simulink model "avionic"  (R2021b)
settings: Solver=ode1  StartTime=0.0  StopTime=inf  FixedStep=0.02  RelTol=1e-3  EnableMultiTasking=on
libraries: bbblueCommlib x13, svdutilitieslib x6, simulink x6, bbblueBasicLib x4, bbblueSensorLib x2
settings Model: ExtModeTrigDuration=100  Creator=ASUS  LastModifiedBy=ASUS
settings SolverCC: PositivePriorityOrder=on  AutoInsertRateTranBlk=on
settings OptimizationCC: EnhancedBackFolding=on  PassReuseOutputArgsAs=Individual arguments  ZeroExternalMemoryAtStartup=off  ZeroInternalMemoryAtStartup=off  MaxStackSize=64  OptimizeBlockOrder=speed  DifferentSizesBufferReuse=on  OptimizationCustomize=off  EfficientTunableParamExpr=on
settings DebuggingCC: ParameterTunabilityLossMsg=error
settings HardwareCC: ProdBitPerPointer=32  ProdBitPerSizeT=32  ProdBitPerPtrDiffT=32  ProdLargestAtomicInteger=Long  ProdLargestAtomicFloat=Double  ProdWordSize=32  ProdHWDeviceType=ARM Compatible->ARM Cortex
settings SFSimCC: MATLABDynamicMemAlloc=off
settings RTWCC: Description=Embedded Coder  SystemTargetFile=ert.tlc  HardwareBoard=BeagleBone Blue  TLCOptions="-aInlineSetEventsForThisBaseRateFcn=TLC_FALSE -aSuppressMultiTaskScheduler=TLC_FALSE  -aRateBasedStepFcn=0"  TemplateMakefile=ert_default_tmf  Toolchain=GNU GCC BeagleBone Blue
settings CodeAppCC: ForceParamTrailComments=on  IgnoreCustomStorageClasses=off  OperatorAnnotations=on  SimulinkDataObjDesc=on  SFDataObjDesc=on  InsertBlockDesc=on
settings ERTTargetCC: SupportContinuousTime=on  SupportVariableSizeSignals=on

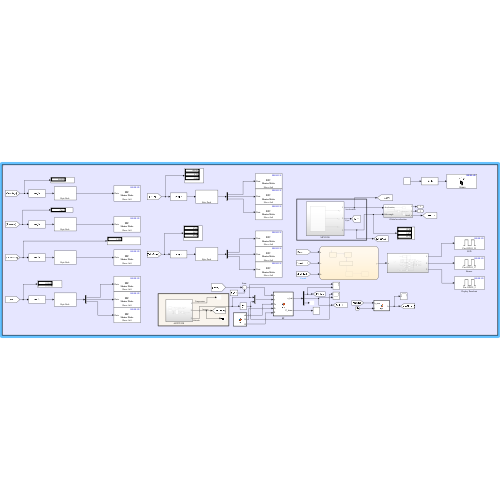
[thumbnail: Simulink's stored preview of the top-level diagram]
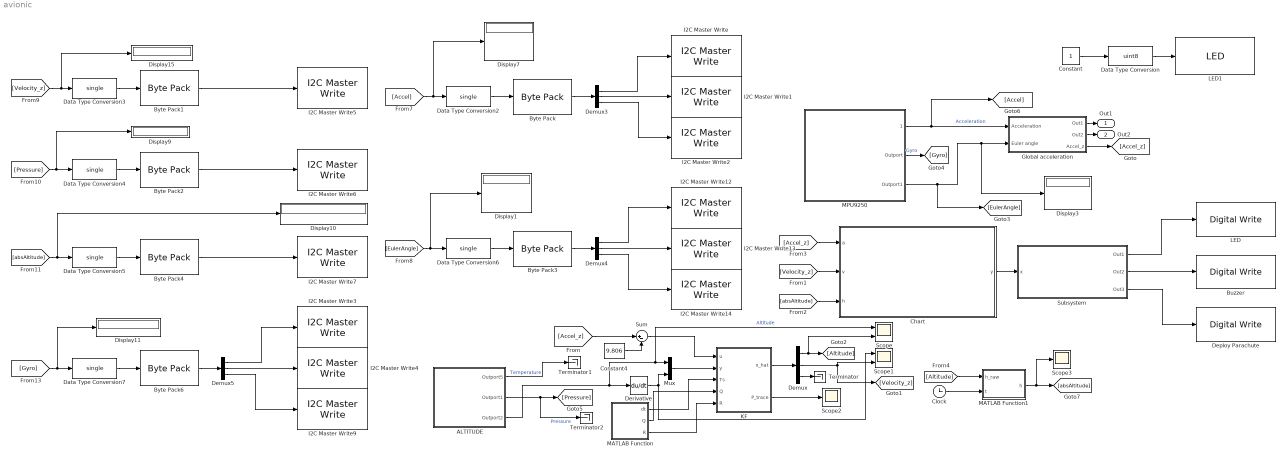
== system avionic ==
  "ALTITUDE " : Subsystem
  "Buzzer " : bbblueBasicLib/Digital Write  GPIOSelect=GPIO1_17  Pin=49  Direction=output
      settings: SourceProductBaseCode=SC_BEAGLEBONE_BLUE
  Byte Pack{,1..4,6} (6 alike) : svdutilitieslib/Byte Pack  maskPackedDataType=uint8  datatypes={'single'}  byteAlign=1  blockPlatform=arduinoert
      settings: SourceProductBaseCode=ANDROID,ARDUINO,ML_ARDUINO,ECCORTEXA,ECCORTEXR,SC_BEAGLEBONE_BLUE,EC_FREEDOM_BOARD,EC_FRDM_K64F,INTEL_BLOCKSET,MICROBIT,NUCLEO,NVIDIA,PX4AUTOPILOTS,RASPPIIO,STMICRODIS,TIC2000,XILINX_BLOCKSET
  Chart : Stateflow chart  TreatAsAtomicUnit=on
  Clock : Clock
  Constant : Constant
  Constant4 : Constant  Value=9.806
  Data Type Conversion : DataTypeConversion  OutDataTypeStr=uint8
  Data Type Conversion{2..7} (6 alike) : DataTypeConversion  OutDataTypeStr=single
  Demux{,3..5} (4 alike) : Demux  Outputs=3
  Deploy Parachute : bbblueBasicLib/Digital Write  GPIOSelect=GPIO3_2  Pin=49  Direction=output
      settings: SourceProductBaseCode=SC_BEAGLEBONE_BLUE
  Derivative : Derivative
  Display{1,3,7,9..11,15} (7 alike) : Display
  Global acceleration : Subsystem
  I2C Master Write{,1..7,9,12..14} (12 alike) : bbblueCommlib/I2C Master Write  I2CModule=1  Mode=Master  SlaveAddress=8  SlaveByteOrder=BigEndian  Direction=Transmitter  RegisterAddressMode=off  RegisterAddress=0  SlaveDataType=uint8  DataLength=1  NoAck=off  RepeatedStart=off  OutputStatus=off
      settings: SourceProductBaseCode=SC_BEAGLEBONE_BLUE
  KF : MATLAB Function  TreatAsAtomicUnit=on
  "LED " : bbblueBasicLib/Digital Write  GPIOSelect=GPIO1_25  Pin=49  Direction=output
      settings: SourceProductBaseCode=SC_BEAGLEBONE_BLUE
  LED1 : bbblueBasicLib/LED  LED=Green
      settings: SourceProductBaseCode=SC_BEAGLEBONE_BLUE
  MATLAB Function : MATLAB Function  TreatAsAtomicUnit=on
  MATLAB Function1 : MATLAB Function  TreatAsAtomicUnit=on
  MPU9250 : Subsystem
  Mux : Mux  Inputs=2
  Scope : Scope  NumInputPorts=2
  Scope1 : Scope  NumInputPorts=2
  Scope2 : Scope
  Scope3 : Scope
  Subsystem : Subsystem
  "Sum " : Sum  Inputs=|+-
  Terminator : Terminator
  Terminator1 : Terminator
  Terminator2 : Terminator
  Out1 : Outport
  Out2 : Outport  Port=2
  wires:
  Demux5/1 -> I2C Master Write3/1
  Subsystem/1(Out1) -> "LED "/1
  MPU9250/1(1) -> [Accel], Global acceleration/1(Acceleration)  "Acceleration"
  Derivative/1 -> Mux/2, Scope1/1
  "ALTITUDE "/3(Outport2) -> Scope/1, Mux/1, Derivative/1  "Altitude"
  [Accel_z] -> "Sum "/1
  "ALTITUDE "/1(Outport5) -> Terminator1/1  "Temperature"
  Data Type Conversion3/1 -> Byte Pack1/1
  Demux3/2 -> I2C Master Write1/1
  Data Type Conversion2/1 -> Byte Pack/1
  Demux4/3 -> I2C Master Write14/1
  Demux3/1 -> I2C Master Write/1
  [Velocity_z] -> Display15/1, Data Type Conversion3/1
  Global acceleration/2(Out2) -> Out2/1
  Byte Pack2/1 -> I2C Master Write6/1
  Demux4/1 -> I2C Master Write12/1
  "ALTITUDE "/2(Outport1) -> [Pressure], Terminator2/1  "Pressure"
  Demux5/2 -> I2C Master Write4/1
  Data Type Conversion6/1 -> Byte Pack3/1
  [Gyro] -> Display11/1, Data Type Conversion7/1
  [EulerAngle] -> Display1/1, Data Type Conversion6/1
  Byte Pack4/1 -> I2C Master Write7/1
  [Velocity_z] -> Chart/2(v)
  Data Type Conversion4/1 -> Byte Pack2/1
  Global acceleration/1(Out1) -> Out1/1
  MPU9250/3(Outport1) -> [EulerAngle], Display3/1, Global acceleration/2(Euler angle)
  Byte Pack1/1 -> I2C Master Write5/1
  Subsystem/3(Out3) -> Deploy Parachute/1
  Data Type Conversion7/1 -> Byte Pack6/1
  Global acceleration/3(Accel_z) -> [Accel_z]
  [absAltitude] -> Display10/1, Data Type Conversion5/1
  Subsystem/2(Out2) -> "Buzzer "/1
  Byte Pack/1 -> Demux3/1
  Demux4/2 -> I2C Master Write13/1
  [Accel_z] -> Chart/1(a)
  [Accel] -> Display7/1, Data Type Conversion2/1
  Demux3/3 -> I2C Master Write2/1
  MPU9250/2(Outport) -> [Gyro]  "Gyro"
  [absAltitude] -> Chart/3(h)
  Chart/1(y) -> Subsystem/1(x)
  Byte Pack3/1 -> Demux4/1
  Byte Pack6/1 -> Demux5/1
  [Pressure] -> Display9/1, Data Type Conversion4/1
  Data Type Conversion5/1 -> Byte Pack4/1
  Demux5/3 -> I2C Master Write9/1
  Data Type Conversion/1 -> LED1/1
  Constant/1 -> Data Type Conversion/1
  Constant4/1 -> "Sum "/2
  "Sum "/1 -> KF/1(u)
  Mux/1 -> KF/2(y)
  MATLAB Function/1(dt) -> KF/3(Ts)
  MATLAB Function/2(Q) -> KF/4(Q)
  MATLAB Function/3(R) -> KF/5(R)
  KF/1(x_hat) -> Demux/1
  KF/2(P_trace) -> Scope2/1
  Demux/1 -> Scope/2, [Altitude]
  Demux/2 -> Scope1/2, [Velocity_z]
  Demux/3 -> Terminator/1
  [Altitude] -> MATLAB Function1/1(h_raw)
  Clock/1 -> MATLAB Function1/2(t)
  MATLAB Function1/1(h) -> Scope3/1, [absAltitude]

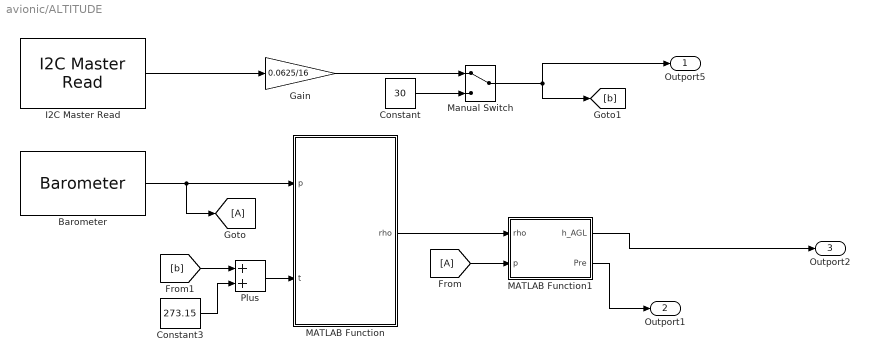
== system avionic/ALTITUDE  ==
  Barometer : bbblueSensorLib/Barometer  OSRSelection=16  IIRFilterCoeff=16  SampleTime=0.02
      settings: SourceProductBaseCode=SC_BEAGLEBONE_BLUE
  Constant : Constant  Value=30
  Constant3 : Constant  Value=273.15
  Gain : Gain  Gain=0.0625/16  OutDataTypeStr=single
  I2C Master Read : bbblueCommlib/I2C Master Read  I2CModule=1  Mode=Master  SlaveAddress=hex2dec('48')  SlaveByteOrder=BigEndian  Direction=Receiver  RegisterAddressMode=off  RegisterAddress=0  SlaveDataType=int16  DataLength=1  NoAck=off  RepeatedStart=off  OutputStatus=off  SampleTime=0.02
      settings: SourceProductBaseCode=SC_BEAGLEBONE_BLUE
  MATLAB Function : MATLAB Function  TreatAsAtomicUnit=on
  MATLAB Function1 : MATLAB Function  TreatAsAtomicUnit=on
  Manual Switch : ManualSwitch
  Plus : Sum
  Outport5 : Outport
  Outport1 : Outport  Port=2
  Outport2 : Outport  Port=3
  wires:
  I2C Master Read/1 -> Gain/1
  Plus/1 -> MATLAB Function/2(t)
  Barometer/1 -> [A], MATLAB Function/1(p)
  Gain/1 -> Manual Switch/1
  MATLAB Function/1(rho) -> MATLAB Function1/1(rho)
  Constant3/1 -> Plus/2
  [A] -> MATLAB Function1/2(p)
  [b] -> Plus/1
  MATLAB Function1/1(h_AGL) -> Outport2/1
  MATLAB Function1/2(Pre) -> Outport1/1
  Constant/1 -> Manual Switch/2
  Manual Switch/1 -> [b], Outport5/1

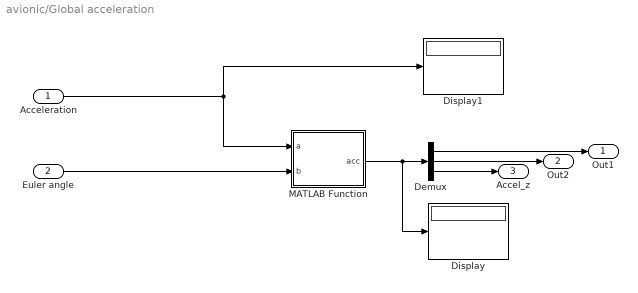
== system avionic/Global acceleration ==
  Acceleration : Inport
  Euler angle : Inport  Port=2
  Demux : Demux  Outputs=3
  Display : Display
  Display1 : Display
  MATLAB Function : MATLAB Function  TreatAsAtomicUnit=on
  Out1 : Outport
  Out2 : Outport  Port=2
  Accel_z : Outport  Port=3
  wires:
  Acceleration/1 -> MATLAB Function/1(a), Display1/1
  MATLAB Function/1(acc) -> Display/1, Demux/1
  Demux/1 -> Out1/1
  Demux/3 -> Accel_z/1
  Euler angle/1 -> MATLAB Function/2(b)
  Demux/2 -> Out2/1

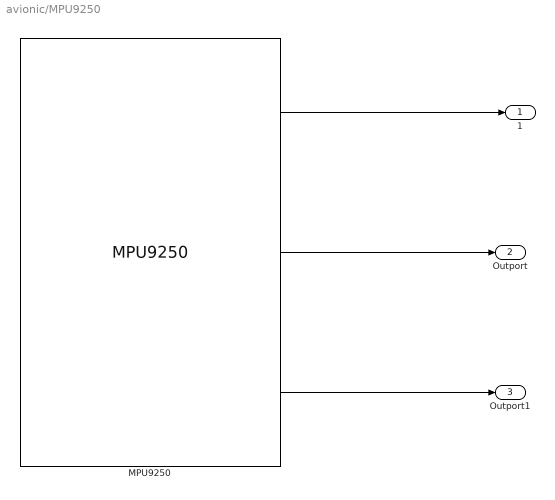
== system avionic/MPU9250 ==
  MPU9250 : bbblueSensorLib/MPU9250  OperationMode=DMP  Accel=on  AngularRate=on  Ak8963Field=off  EulerAngles=on  Quat=off  AccelRange=16G  Acceldlpf=1  GyroRange=250 dps  Gyrodlpf=1  DmpOdr=200 Hz  SampleTime=0.02
      settings: SourceProductBaseCode=SC_BEAGLEBONE_BLUE
  1 : Outport
  Outport : Outport  Port=2
  Outport1 : Outport  Port=3
  wires:
  MPU9250/1 -> 1/1
  MPU9250/2 -> Outport/1
  MPU9250/3 -> Outport1/1

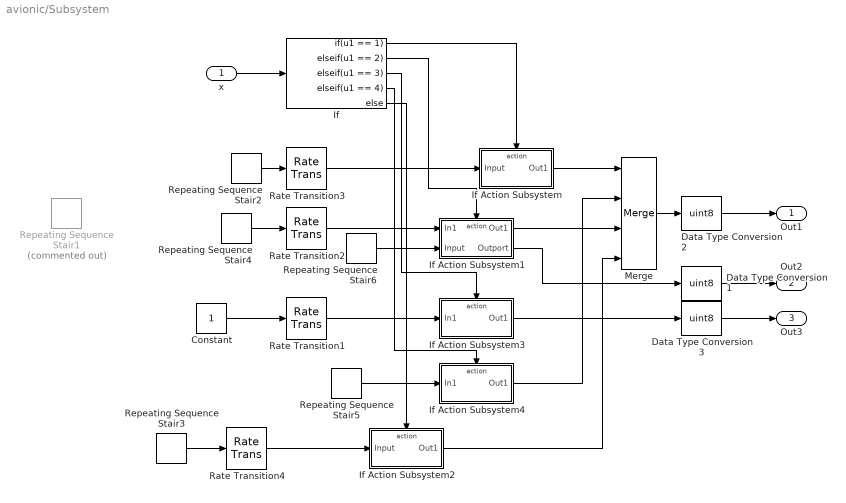
== system avionic/Subsystem ==
  x : Inport
  Constant : Constant
  Data Type Conversion1 : DataTypeConversion  OutDataTypeStr=uint8
  Data Type Conversion2 : DataTypeConversion  OutDataTypeStr=uint8
  Data Type Conversion3 : DataTypeConversion  OutDataTypeStr=uint8
  If : If  IfExpression=u1 == 1  ElseIfExpressions=u1 == 2, u1 == 3, u1 == 4
  If Action Subsystem : Subsystem  TreatAsAtomicUnit=on
  If Action Subsystem1 : Subsystem  TreatAsAtomicUnit=on
  If Action Subsystem2 : Subsystem  TreatAsAtomicUnit=on
  If Action Subsystem3 : Subsystem  TreatAsAtomicUnit=on
  If Action Subsystem4 : Subsystem  TreatAsAtomicUnit=on
  Merge : Merge  Inputs=4
  Rate Transition{1..4} (4 alike) : RateTransition
  Repeating Sequence Stair1 : simulink/Sources/Repeating Sequence Stair  Commented=on  OutValues=[1 0 1 0 0 0 0 0].'  tsamp=0.1  OutMin=[]  OutMax=[]  OutDataTypeStr=double  OutputDataTypeScalingMode=double  OutDataType=fixdt(0,8)  ConRadixGroup=Best Precision: Vector-wise  OutScaling=2^-12
  Repeating Sequence Stair2 : simulink/Sources/Repeating Sequence Stair  OutValues=[1 1 1 1 1 0 0 0 0 0].'  tsamp=0.1  OutMin=[]  OutMax=[]  OutDataTypeStr=double  OutputDataTypeScalingMode=double  OutDataType=fixdt(0,8)  ConRadixGroup=Best Precision: Vector-wise  OutScaling=2^-12
  Repeating Sequence Stair3 : simulink/Sources/Repeating Sequence Stair  OutValues=[1 0 0 0 0 0 0 0 0 0 0 0 0 0 0 0].'  tsamp=0.1  OutMin=[]  OutMax=[]  OutDataTypeStr=double  OutputDataTypeScalingMode=double  OutDataType=fixdt(0,8)  ConRadixGroup=Best Precision: Vector-wise  OutScaling=2^-12
  Repeating Sequence Stair4 : simulink/Sources/Repeating Sequence Stair  OutValues=[1 0 1 0 1 0 0 0].'  tsamp=0.1  OutMin=[]  OutMax=[]  OutDataTypeStr=double  OutputDataTypeScalingMode=double  OutDataType=fixdt(0,8)  ConRadixGroup=Best Precision: Vector-wise  OutScaling=2^-12
  Repeating Sequence Stair5 : simulink/Sources/Repeating Sequence Stair  OutValues=[1 0 1 0 0 0 0 0].'  tsamp=0.1  OutMin=[]  OutMax=[]  OutDataTypeStr=double  OutputDataTypeScalingMode=double  OutDataType=fixdt(0,8)  ConRadixGroup=Best Precision: Vector-wise  OutScaling=2^-12
  Repeating Sequence Stair6 : simulink/Sources/Repeating Sequence Stair  OutValues=[1 0 1 0 1 0 0 0].'  tsamp=0.5  OutMin=[]  OutMax=[]  OutDataTypeStr=double  OutputDataTypeScalingMode=double  OutDataType=fixdt(0,8)  ConRadixGroup=Best Precision: Vector-wise  OutScaling=2^-12
  Out1 : Outport
  Out2 : Outport  Port=2
  Out3 : Outport  Port=3
  wires:
  If/5 -> If Action Subsystem2/Action
  If/1 -> If Action Subsystem/Action
  Repeating Sequence Stair4/1 -> Rate Transition2/1
  Rate Transition2/1 -> If Action Subsystem1/1(In1)
  Merge/1 -> Data Type Conversion2/1
  If Action Subsystem/1(Out1) -> Merge/1
  If Action Subsystem1/1(Out1) -> Merge/3
  If/2 -> If Action Subsystem1/Action
  Data Type Conversion2/1 -> Out1/1
  x/1 -> If/1
  Constant/1 -> Rate Transition1/1
  Rate Transition1/1 -> If Action Subsystem3/1(In1)
  If/3 -> If Action Subsystem3/Action
  If Action Subsystem4/1(Out1) -> Merge/2
  Repeating Sequence Stair5/1 -> If Action Subsystem4/1(In1)
  If/4 -> If Action Subsystem4/Action
  Repeating Sequence Stair2/1 -> Rate Transition3/1
  Rate Transition3/1 -> If Action Subsystem/1(Input)
  Data Type Conversion1/1 -> Out2/1
  Repeating Sequence Stair6/1 -> If Action Subsystem1/2(Input)
  If Action Subsystem1/2(Outport) -> Data Type Conversion1/1
  Repeating Sequence Stair3/1 -> Rate Transition4/1
  Rate Transition4/1 -> If Action Subsystem2/1(Input)
  If Action Subsystem3/1(Out1) -> Data Type Conversion3/1
  If Action Subsystem2/1(Out1) -> Merge/4
  Data Type Conversion3/1 -> Out3/1

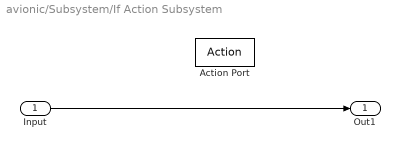
== system avionic/Subsystem/If Action Subsystem ==
  Input : Inport
  Action Port : ActionPort  ActionPortLabel=if(u1 == 1)
  Out1 : Outport
  wires:
  Input/1 -> Out1/1

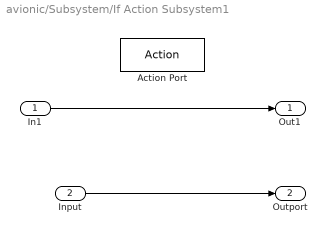
== system avionic/Subsystem/If Action Subsystem1 ==
  In1 : Inport
  Input : Inport  Port=2
  Action Port : ActionPort  ActionPortLabel=elseif(u1 == 2)
  Out1 : Outport
  Outport : Outport  Port=2
  wires:
  In1/1 -> Out1/1
  Input/1 -> Outport/1

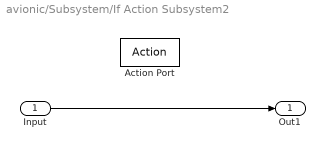
== system avionic/Subsystem/If Action Subsystem2 ==
  Input : Inport
  Action Port : ActionPort  ActionPortLabel=else
  Out1 : Outport
  wires:
  Input/1 -> Out1/1

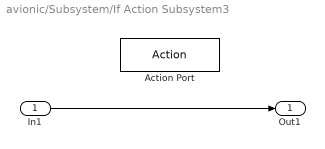
== system avionic/Subsystem/If Action Subsystem3 ==
  In1 : Inport
  Action Port : ActionPort  ActionPortLabel=elseif( u1 == 3)
  Out1 : Outport
  wires:
  In1/1 -> Out1/1

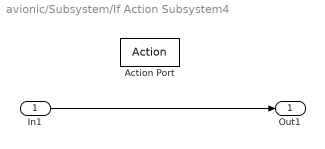
== system avionic/Subsystem/If Action Subsystem4 ==
  In1 : Inport
  Action Port : ActionPort  ActionPortLabel=elseif( u1 == 4)
  Out1 : Outport
  wires:
  In1/1 -> Out1/1

== matlab function avionic/MATLAB Function ==
  data: dt output; Q output; R output
function [dt,Q,R] = fcn

%n  = 3;
dt = 0.02;

Q = 1e-8*diag([1 1 10000]);
R = 1e1*diag([1 40]);

== matlab function avionic/Global acceleration/MATLAB Function ==
  data: a input; acc output; b input
function acc = fcn(a,b)
b1= b(1)*pi/180; %roll
b2 = b(2)*pi/180; %pitch
b3 = b(3)*pi/180; %yaw
Rz = [cos(b3) sin(b3) 0 ;
    -sin(b3) cos(b3) 0;
    0 0 1];

Rx = [1 0 0;
    0 cos(b1) sin(b1);
    0 -sin(b1) cos(b1)];

Ry = [cos(b2) 0 -sin(b2);
    0 1 0;
    sin(b2) 0 cos(b2)];

acc = (Rx*Ry*Rz)'*a;

== stateflow chart avionic/Chart ==
  state OnLaunchPad
    y=0;
    y=2;
  state LaunchDetect
    y=1;
  state ApogeeDetect
    y=3;
  state Droping [commented out]
    y=3;
  state TouchDown [commented out]
    y=4;
  (default) -> OnLaunchPad
  OnLaunchPad -> LaunchDetect : [a>9.81*3]
  LaunchDetect -> ApogeeDetect : [v<=1 & h>50]
  ApogeeDetect -> Droping [commented out] : after(3,sec)
  Droping -> TouchDown [commented out] : [abs(a)>5*9.81]
  data: a input; y output; v input; h input

== matlab function avionic/MATLAB Function1 ==
  data: h_raw input; h output; t input
function h = fcn(h_raw, t)

persistent h_offset
if isempty(h_offset), h_offset = h_raw; end
if t<3
    h_offset = h_raw;
end

h = h_raw - h_offset;

== matlab function avionic/ALTITUDE /MATLAB Function ==
  data: p input; rho output; t input
function rho = fcn(p,t)

M = 0.0289644; %kg/mol\
R = 8.31432; %Nm/molK

rho = (M*p)/(R*t);

== matlab function avionic/KF ==
  settings: updateMethod=DISCRETE
  data: u input; x_hat output; P_trace output; y input; Ts input; Q input; R input
function [x_hat,P_trace] = fcn(u,y,Ts,Q,R)

persistent x_ P_
if isempty(x_), x_= [0;0;0.1]; P_ = 1e0*diag([1 1 100]);end

% a_IMU = a - ba
% v_dot = a
% h_dot = v
% let x1 = h, x2 = v, x3 = ba
% x1_dot = x2
% x2_dot = a_IMU + x3
% x3_dot = 0

A = [0  1   0
     0  0   1
     0  0   0];
B = [0;1;0];
Ad = eye(3) + A*Ts;
Bd = B*Ts;

x = Ad*x_ + Bd*u; 
P = Ad*P_*Ad'+ Q;

C = [1 0 0
     0 1 0];
W = (P*C')/(C*P*C'+ R);
x = x + W*(y(1:2,1)-C*x);
P = P - W*C*P;

x_hat = x;
P_trace = trace(P);
x_ = x;
P_ = P;

== matlab function avionic/ALTITUDE /MATLAB Function1 ==
  data: rho input; h_AGL output; p input; Pre output
function [h_AGL, Pre]= fcn(rho,p)
P0 = 101325; %N/m^2
g = 9.80665; %m/s^2
hg = 14.3256; %m 
Pre = p-P0;
h = (Pre)/-(rho*g);
h_AGL = h-hg
